simulink model "MCuC"  (R2023b)
settings: Solver=ode8  StartTime=0.0  StopTime=10.0  FixedStep=.0001  RelTol=1e-3
settings Model: DataDictionary=rev3_data.sldd  Creator=mjmag  LastModifiedBy=mjmag

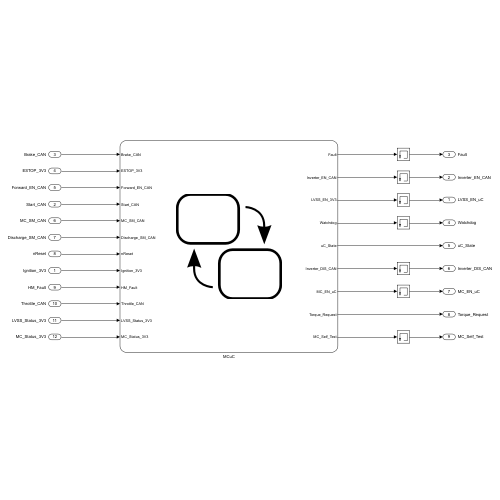
[thumbnail: Simulink's stored preview of the top-level diagram]
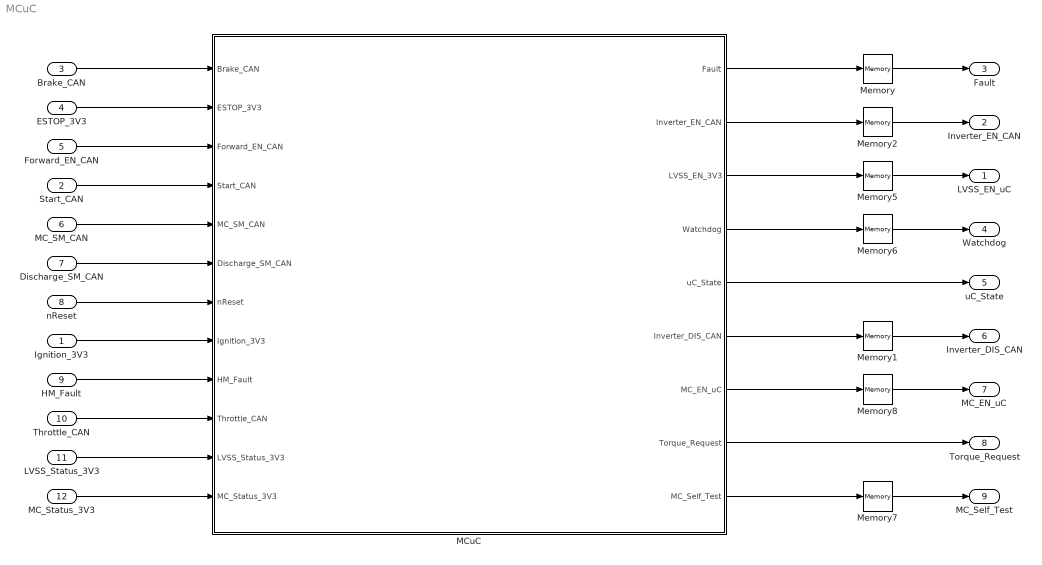
== system MCuC ==
  Ignition_3V3 : Inport  OutDataTypeStr=boolean
  Start_CAN : Inport  Port=2  OutDataTypeStr=boolean
  Brake_CAN : Inport  Port=3  OutDataTypeStr=boolean
  ESTOP_3V3 : Inport  Port=4  OutDataTypeStr=boolean
  Forward_EN_CAN : Inport  Port=5  OutDataTypeStr=boolean
  MC_SM_CAN : Inport  Port=6  OutDataTypeStr=Enum: MC_VSM_State
  Discharge_SM_CAN : Inport  Port=7  OutDataTypeStr=Enum: MC_DC_State
  nReset : Inport  Port=8  OutDataTypeStr=boolean
  HM_Fault : Inport  Port=9  OutDataTypeStr=boolean
  Throttle_CAN : Inport  Port=10  OutDataTypeStr=int16
  LVSS_Status_3V3 : Inport  Port=11  OutDataTypeStr=boolean
  MC_Status_3V3 : Inport  Port=12  OutDataTypeStr=boolean
  MCuC : Stateflow chart  TreatAsAtomicUnit=on
      settings: PortSchema="{\"entries\":[{\"content\":{\"sides\":[{\"content\":{\"connectorIds\":[\"In1\",\"In2\",\"In3\",\"In5\",\"In6\",\"In7\",\"In8\",\"In4\",\"In9\",\"In10\",\"In11\",\"In12\"]},\"type\":\"ConnectorPlacement.EquallySpacedRectSide\",\"uuid\":\"d1510c73-f1c7-4e03-bb6c-bda7856f993e\"},{\"content\":{\"connectorIds\":[\"Out1\",\"Out2\",\"Out3\",\"Out4\",\"Out5\",\"Out6\",\"Out7\",\"Out8\",\"Out9\"],\"side\":\"RIGHT\"},\"type\":\"ConnectorPlacement.EquallySpacedRectSide\",\"uuid\":\"1a7878c4-a817-4ca0-b21c-0429e82bb9d7\"},{\"content\":{\"side\":\"TOP\"},\"type\":\"ConnectorPlacement.EquallySpacedRectSide\",\"uuid\":\"ed9f2701-7044-4bb4-9c0b-b9cf9840e69e\"}]},\"type\":\"ConnectorPlacement.EquallySpacedConnector\",\"uuid\":\"4ceb8e7d-629c-4438-88a9-aa3016537644\"}],\"packageUris\":[\"http://schema.mathworks.com/mf0/Connector/R2020b\"],\"version\":\"1.0\"}"
  Memory{,1..2,5..8} (7 alike) : Memory
  LVSS_EN_uC : Outport  OutDataTypeStr=boolean
  Inverter_EN_CAN : Outport  Port=2
  Fault : Outport  Port=3
  Watchdog : Outport  Port=4  OutDataTypeStr=boolean
  uC_State : Outport  Port=5  OutDataTypeStr=Enum: UC_State
  Inverter_DIS_CAN : Outport  Port=6
  MC_EN_uC : Outport  Port=7  OutDataTypeStr=boolean
  Torque_Request : Outport  Port=8  OutDataTypeStr=int16
  MC_Self_Test : Outport  Port=9
  wires:
  MCuC/1(Fault) -> Memory/1
  MCuC/9(MC_Self_Test) -> Memory7/1
  MCuC/5(uC_State) -> uC_State/1
  Memory7/1 -> MC_Self_Test/1
  MCuC/3(LVSS_EN_3V3) -> Memory5/1
  Memory1/1 -> Inverter_DIS_CAN/1
  Memory5/1 -> LVSS_EN_uC/1
  Memory2/1 -> Inverter_EN_CAN/1
  Memory/1 -> Fault/1
  Memory8/1 -> MC_EN_uC/1
  Memory6/1 -> Watchdog/1
  MCuC/7(MC_EN_uC) -> Memory8/1
  Ignition_3V3/1 -> MCuC/4(Ignition_3V3)
  ESTOP_3V3/1 -> MCuC/2(ESTOP_3V3)
  Start_CAN/1 -> MCuC/5(Start_CAN)
  Brake_CAN/1 -> MCuC/1(Brake_CAN)
  Forward_EN_CAN/1 -> MCuC/3(Forward_EN_CAN)
  Throttle_CAN/1 -> MCuC/10(Throttle_CAN)
  MC_SM_CAN/1 -> MCuC/6(MC_SM_CAN)
  Discharge_SM_CAN/1 -> MCuC/7(Discharge_SM_CAN)
  nReset/1 -> MCuC/8(nReset)
  HM_Fault/1 -> MCuC/9(HM_Fault)
  LVSS_Status_3V3/1 -> MCuC/11(LVSS_Status_3V3)
  MC_Status_3V3/1 -> MCuC/12(MC_Status_3V3)
  MCuC/4(Watchdog) -> Memory6/1
  MCuC/2(Inverter_EN_CAN) -> Memory2/1
  MCuC/6(Inverter_DIS_CAN) -> Memory1/1
  MCuC/8(Torque_Request) -> Torque_Request/1

== stateflow chart MCuC/MCuC ==
  state MCuC
    state MCuC_Logic [parallel]
      settings: executionOrder=1
      state MC_Off
        entry:
        LVSS_EN_3V3 = false;
        uC_State = UC_State.MC_Off;
        uncharged = true;
        Inverter_EN_CAN = false;
      state LVSS_MC_Shutdown
        entry:
        uC_State = UC_State.LVSS_MC_Shutdown;
        LVSS_EN_3V3 = false;
        Inverter_DIS_CAN = false;
        MC_EN_uC = false;
      state MC_Discharging
        entry:
        uC_State = UC_State.MC_Discharging;
      state ESTOP
        entry:
        uC_State = UC_State.Estop;
        LVSS_EN_3V3 = false;
        ESTOP_activated = false;
      state Fault_Ignit_H
      state LVSS_MC_Startup
        entry:
        uncharged = false;
        uC_State = UC_State.LVSS_MC_Startup;
        LVSS_EN_3V3 = true;
        MC_EN_uC = true;
      state Fault
        entry:
        uC_State = UC_State.Fault;
        Fault_Activated = false;
        Fault = true;
        exit:
        Fault = false;
      state Contactor_Open
        entry:
        Inverter_EN_CAN = false;
        Inverter_DIS_CAN = true;
        uC_State = UC_State.Contactor_Open;
      state MC_Init
        entry:
        uC_State = UC_State.MC_Init;
      state Preset
        entry:
        uC_State = UC_State.Preset;
        state MC_ST
          entry:
          MC_Self_Test = true
          state MC_EN_ON
            entry:
            MC_EN_uC = true;
          state MC_EN_OFF
            entry:
            MC_EN_uC = false;
          (default) -> MC_EN_ON
          MC_EN_ON -> MC_EN_OFF : [MC_Status_3V3 == true]
        (default) -> MC_ST
      state Contactor_Closed
        entry:
        uC_State = UC_State.Contactor_Closed;
        Inverter_EN_CAN = false;
      state MC_Active
        entry:
        Inverter_EN_CAN = true;
        uC_State = UC_State.MC_Active;
        Torque_Request = 0;
        during:
        Torque_Request = Throttle_CAN;
        exit:
        Torque_Request = 0;
      LVSS_MC_Shutdown -> MC_Off : [MC_Status_3V3 == false && LVSS_Status_3V3 == false]
      Fault_Ignit_H -> MC_Off : [Ignition_3V3 == false]
      MC_Discharging -> LVSS_MC_Shutdown : [Discharge_SM_CAN == MC_DC_State.Complete]
      MCuC_Logic -> ESTOP [order 3] : [ESTOP_3V3 == true && uncharged == true && nReset == true && uC_State ~= UC_State.Preset]
      ESTOP -> MC_Off : [ESTOP_3V3 == false]
      Preset -> MC_Off : [MC_Status_3V3 == false && Ignition_3V3 == false && LVSS_Status_3V3 == false]
          | {MC_Self_Test = false}
      MC_Off -> LVSS_MC_Startup : [Ignition_3V3 == true]
      Contactor_Open -> MC_Discharging : [Discharge_SM_CAN ~= MC_DC_State.Disabled]
      Fault -> Fault_Ignit_H : [MC_Status_3V3 == false && Ignition_3V3 == true]
      MCuC_Logic -> Fault [order 4] : [HM_Fault == true && uncharged == true && uC_State ~= UC_State.Preset && nReset == true]
      LVSS_MC_Startup -> MC_Init : [MC_Status_3V3 == true && LVSS_Status_3V3 == true]
      (default) -> Preset
      MCuC_Logic -> Contactor_Open [order 1] : [HM_Fault == true && Ignition_3V3 == true && uncharged == false && Fault_Activated == false]{Fault_Activated = true}
      MCuC_Logic -> Contactor_Open [order 2] : [ESTOP_3V3 == true && uncharged == false && ESTOP_activated == false]{ESTOP_activated = true}
      MCuC_Logic -> Preset [order 5] : [nReset == false]
      MC_Init -> Contactor_Open [order 1] : [Ignition_3V3 == false]
      Contactor_Closed -> Contactor_Open [order 2] : [Ignition_3V3 == false]
      MC_Active -> Contactor_Open [order 2] : [Ignition_3V3 == false]
      MC_Init -> Contactor_Closed [order 2] : [MC_SM_CAN == MC_VSM_State.Ready]
      Contactor_Closed -> MC_Active [order 1] : [Start_CAN == true && Forward_EN_CAN == true && Brake_CAN == true && Throttle_CAN == 0]
      MC_Active -> Contactor_Closed [order 1] : [Forward_EN_CAN == false]
    state Watchdog [parallel]
      settings: executionOrder=2
      state WD0
        entry:
        Watchdog = false;
      state WD1
        entry:
        Watchdog = true;
      (default) -> WD0
      WD0 -> WD1 : after(.5, sec)
      WD1 -> WD0 : after(.5, sec)
  data: Fault output =false; Brake_CAN input; ESTOP_3V3 input; Forward_EN_CAN input; Ignition_3V3 input; Start_CAN input; MC_SM_CAN input; Inverter_EN_CAN output =false; LVSS_EN_3V3 output =false; Discharge_SM_CAN input; nReset input; Watchdog output =false; uC_State output =UC_State.MC_Off; uncharged local =true; ESTOP_activated local =false; HM_Fault input; Throttle_CAN input; Inverter_DIS_CAN output =false; MC_EN_uC output =false; LVSS_Status_3V3 input; MC_Status_3V3 input; Torque_Request output int16 =0; Fault_Activated local =false; MC_Self_Test output
